simulink model "motor_pos_sensor_Harness1"  (R2023a)
settings: configuration reference "config" (kept outside this file)
libraries: simulink x1
settings Model: DataDictionary=model_config.sldd  Creator=Administrator  LastModifiedBy=Administrator
settings ConfigSetRef: SourceName=config

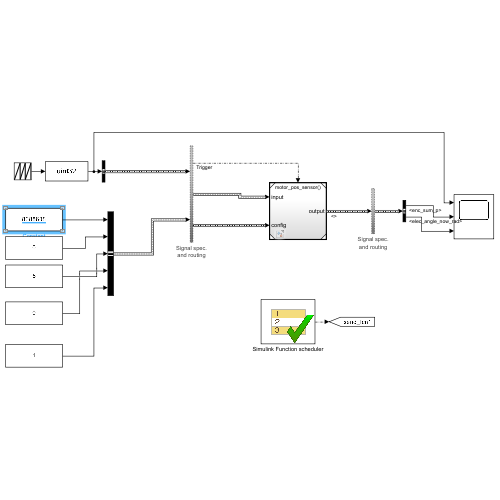
[thumbnail: Simulink's stored preview of the top-level diagram]
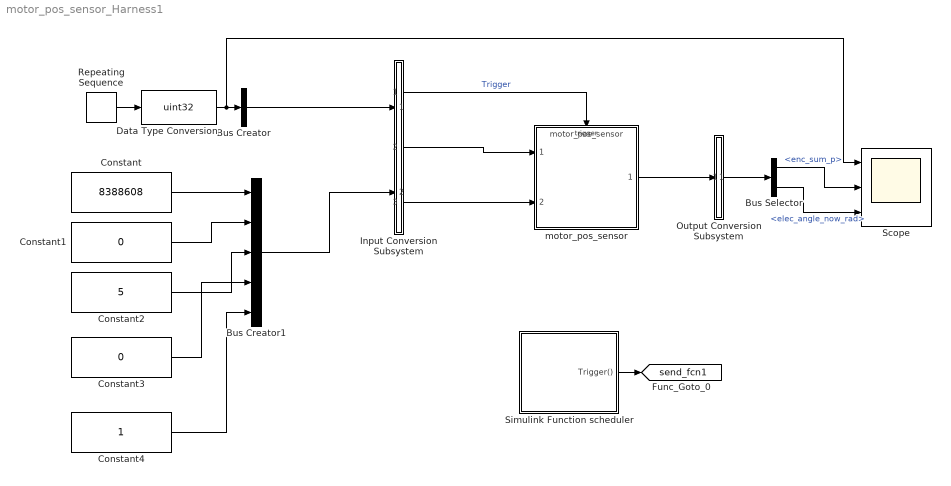
== system motor_pos_sensor_Harness1 ==
  Bus Creator : BusCreator  Inputs=1  OutDataTypeStr=Bus: MotorPosSensorInput  NonVirtualBus=on
      settings: InheritFromInputs=off
  Bus Creator1 : BusCreator  Inputs=5  OutDataTypeStr=Bus: MotorPosSensorConfig  NonVirtualBus=on
      settings: InheritFromInputs=off
  Bus Selector : BusSelector  OutputSignals=enc_sum_p,elec_angle_now_rad
  Constant : Constant  Value=8388608  OutDataTypeStr=uint32
  Constant1 : Constant  Value=0  OutDataTypeStr=int64
  Constant2 : Constant  Value=5  OutDataTypeStr=uint32
  Constant3 : Constant  Value=0  OutDataTypeStr=single
  Constant4 : Constant  OutDataTypeStr=int8
  Data Type Conversion : DataTypeConversion  OutDataTypeStr=uint32  SaturateOnIntegerOverflow=off  RndMeth=Floor
  Input Conversion Subsystem : Subsystem  Tag=__SLT_ICS__  Description=|
      | Signal spec.
      | and routing
      settings: AttributesFormatString=%<Description>
  Output Conversion Subsystem : Subsystem  Tag=__SLT_OCS__  Description=|
      | Signal spec.
      | and routing
      settings: AttributesFormatString=%<Description>
  Repeating Sequence : simulink/Sources/Repeating Sequence  rep_seq_t=[0 1]  rep_seq_y=[0 8388607]
  Scope : Scope  NumInputPorts=3
  Simulink Function scheduler : Test Sequence  Tag=__SLT_FCN_CALL__  TreatAsAtomicUnit=on
  motor_pos_sensor : ModelReference  ModelNameDialog=motor_pos_sensor  SimulationMode=Normal  ModelReferenceVersion=2.957  TriggerPortName=Trigger  TriggerPortTriggerType=function-call  TriggerPortStatesWhenEnabling=held
  tag scope: send_fcn1=global
  wires:
  Input Conversion Subsystem/2(Outport_1) -> motor_pos_sensor/1
  Input Conversion Subsystem/3(Outport_2) -> motor_pos_sensor/2
  motor_pos_sensor/1 -> Output Conversion Subsystem/1(Inport_1)
  Simulink Function scheduler/1(Trigger()) -> [send_fcn1]
  Repeating Sequence/1 -> Data Type Conversion/1
  Bus Creator/1 -> Input Conversion Subsystem/1(Inport_1)
  Constant/1 -> Bus Creator1/1
  Constant1/1 -> Bus Creator1/2
  Constant2/1 -> Bus Creator1/3
  Constant3/1 -> Bus Creator1/4
  Constant4/1 -> Bus Creator1/5
  Bus Creator1/1 -> Input Conversion Subsystem/2(Inport_2)
  Output Conversion Subsystem/1(Outport_1) -> Bus Selector/1
  Bus Selector/1 -> Scope/2  "<enc_sum_p>"
  Bus Selector/2 -> Scope/3  "<elec_angle_now_rad>"
  Data Type Conversion/1 -> Scope/1, Bus Creator/1
  Input Conversion Subsystem/1(Outport_3) -> motor_pos_sensor/Trigger  "Trigger"

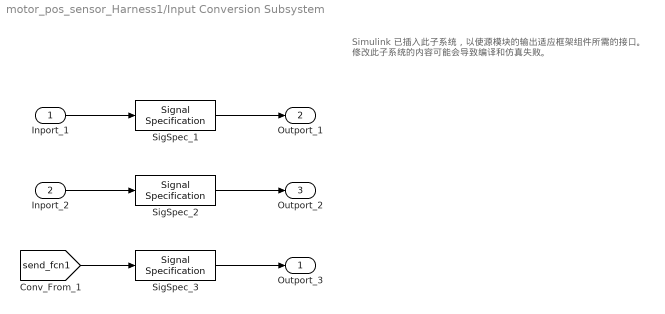
== system motor_pos_sensor_Harness1/Input Conversion Subsystem ==
  note: Simulink 已插入此子系统，以使源模块的输出适应框架组件所需的接口。
      |  修改此子系统的内容可能会导致编译和仿真失败。
  Inport_1 : Inport
  Inport_2 : Inport  Port=2
  SigSpec_1 : SignalSpecification  OutDataTypeStr=Bus: MotorPosSensorInput  Dimensions=[1]  BusOutputAsStruct=on
  SigSpec_2 : SignalSpecification  OutDataTypeStr=Bus: MotorPosSensorConfig  Dimensions=[1]  BusOutputAsStruct=on
  SigSpec_3 : SignalSpecification
  Outport_3 : Outport
  Outport_1 : Outport  Port=2
  Outport_2 : Outport  Port=3
  wires:
  SigSpec_1/1 -> Outport_1/1
  Inport_1/1 -> SigSpec_1/1
  SigSpec_2/1 -> Outport_2/1
  Inport_2/1 -> SigSpec_2/1
  SigSpec_3/1 -> Outport_3/1
  [send_fcn1] -> SigSpec_3/1

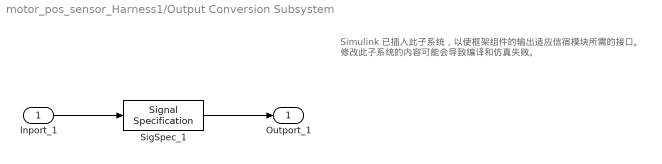
== system motor_pos_sensor_Harness1/Output Conversion Subsystem ==
  note: Simulink 已插入此子系统，以使框架组件的输出适应信宿模块所需的接口。
      |  修改此子系统的内容可能会导致编译和仿真失败。
  Inport_1 : Inport
  SigSpec_1 : SignalSpecification  OutDataTypeStr=Bus: MotorPosSensorOutput  Dimensions=[1]  BusOutputAsStruct=on
  Outport_1 : Outport
  wires:
  Inport_1/1 -> SigSpec_1/1
  SigSpec_1/1 -> Outport_1/1

== stateflow chart motor_pos_sensor_Harness1/Simulink Function scheduler ==
  settings: updateMethod=DISCRETE  sampleTime=1.0E-5
  state Run
    num = 0;
    send(Trigger);
  state step_1
    num = num +1;
  state step_2
    num = 0;
    send(Trigger);
  (default) -> Run
  Run -> step_1 : [
      | true
      | ]
  step_1 -> step_2 : [
      | num >  8
      | ]
  step_2 -> step_1 : [
      | true
      | ]
  data: num local
  events: Trigger output FUNCTION_CALL_EVENT
